simulink model "ExampleModel"  (R2020b)
settings: Solver=FixedStepAuto  StartTime=0.0  StopTime=10.0  FixedStep=0.010  RelTol=1e-3
libraries: TcSimInterface x1
settings Model: Creator=kaebi  LastModifiedBy=kaebi
settings ConfigComp: PLC_TargetIDE=codesys23

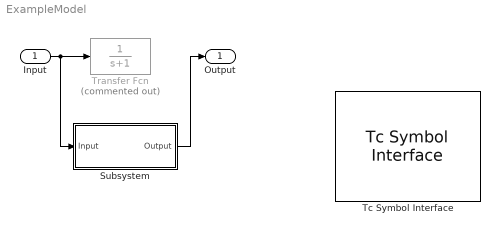
== system ExampleModel ==
  Input : Inport
  Subsystem : Subsystem  TreatAsAtomicUnit=on
  Tc Symbol Interface : TcSimInterface/Tc Symbol Interface  ChangeRowColOrder=on  TraceMode=3  DirectFeedThrough=0  SignalLabels=3  PortLabels=2  ExpandBusObjDepth=on  RuntimeConfig=|  SyncClockMode=1
      | <?xml version="1.0" encoding="UTF-8" standalone="no"?>
      | <TcRuntimAdapterProject>
      | 	<DataTypes/>
      | 	<Translations/>
      | 	<System>
      | 		<Tasks/>
      | 		<Modules/>
      | 	</System>
      | </TcRuntimAdapterProject>
      settings: SourceProductName=Beckhoff TwinCAT Interface
  Transfer Fcn : TransferFcn  Commented=on  Denominator=[1 1]
  Output : Outport
  wires:
  Input/1 -> Transfer Fcn/1, Subsystem/1(Input)
  Subsystem/1(Output) -> Output/1

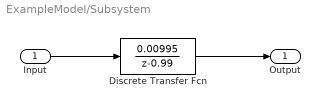
== system ExampleModel/Subsystem ==
  Input : Inport
  Discrete Transfer Fcn : DiscreteTransferFcn  Numerator=[0.00995]  Denominator=[1 -0.99]
  Output : Outport
  wires:
  Input/1 -> Discrete Transfer Fcn/1
  Discrete Transfer Fcn/1 -> Output/1
